simulink model "DEF_Link"  (R2018b)
settings: Solver=FixedStepDiscrete  StartTime=0.0  StopTime=10  FixedStep=0.025  RelTol=1e-3
values from neighbouring files (symbols this model uses):
  Cst_0U = uint8(0)    [DEF_ROM.m]
settings Model: Creator=CKJH7536T  LastModifiedBy=sambit.m
settings DataIOCC: LimitDataPoints=on  SaveFormat=Array  SaveOutput=off  SaveTime=off
settings OptimizationCC: DefaultParameterBehavior=Inlined  UseDivisionForNetSlopeComputation=on  UseFloatMulNetSlope=on  InlineInvariantSignals=on  EnhancedBackFolding=on  PassReuseOutputArgsAs=Individual arguments  ZeroExternalMemoryAtStartup=off  ZeroInternalMemoryAtStartup=off  NoFixptDivByZeroProtection=on  EfficientFloat2IntCast=on  OptimizeBlockOrder=speed  DifferentSizesBufferReuse=on  OptimizationCustomize=off
settings DebuggingCC: ConsistencyChecking=error  SignalInfNanChecking=error  ReadBeforeWriteMsg=EnableAllAsError  WriteAfterWriteMsg=EnableAllAsError  WriteAfterReadMsg=EnableAllAsError  AlgebraicLoopMsg=error  ArtificialAlgebraicLoopMsg=error  SaveWithDisabledLinksMsg=none  MergeDetectMultiDrivingBlocksExec=none  SignalResolutionControl=None  BlockPriorityViolationMsg=error  MinStepSizeMsg=error  TimeAdjustmentMsg=warning  SolverPrmCheckMsg=error  InheritedTsInSrcMsg=error  SingleTaskRateTransMsg=error  TasksWithSamePriorityMsg=error  SigSpecEnsureSampleTimeMsg=error  CheckMatrixSingularityMsg=error  ParameterOverflowMsg=none  ParameterPrecisionLossMsg=none  ParameterTunabilityLossMsg=error  UnderSpecifiedDataTypeMsg=warning  VectorMatrixConversionMsg=error  FcnCallInpInsideContextMsg=warning  SignalLabelMismatchMsg=warning  UnconnectedInputMsg=error  UnconnectedOutputMsg=error  UnconnectedLineMsg=error  SFcnCompatibilityMsg=error  UniqueDataStoreMsg=error  BusObjectLabelMismatch=error  RootOutportRequireBusObject=error  AssertControl=DisableAll  ModelReferenceIOMsg=error  ModelReferenceVersionMismatchMessage=error  ModelReferenceIOMismatchMessage=error  UnknownTsInhSupMsg=error  ModelReferenceDataLoggingMessage=error  StateNameClashWarn=warning  StrictBusMsg=ErrorOnBusTreatedAsVector  NonBusSignalsTreatedAsBus=error  SFInvalidInputDataAccessInChartInitDiag=error  SFTransitionOutsideNaturalParentDiag=error  SFExecutionAtInitializationDiag=none
settings HardwareCC: ProdBitPerPointer=32  ProdBitPerSizeT=32  ProdBitPerPtrDiffT=32  ProdLargestAtomicInteger=Long  ProdLargestAtomicFloat=Double  ProdWordSize=32  ProdLongLongMode=on  ProdHWDeviceType=ARM Compatible->ARM Cortex
settings ModelReferenceCC: PropagateSignalLabelsOutOfModel=off
settings SFSimCC: MATLABDynamicMemAlloc=off
settings RTWCC: SystemTargetFile=ert.tlc  GenCodeOnly=on  TemplateMakefile=ert_default_tmf  GenerateReport=on  IncludeHyperlinkInReport=on  LaunchReport=on  GenerateTraceInfo=on  GenerateTraceReport=on  GenerateTraceReportSl=on  GenerateTraceReportSf=on  GenerateTraceReportEml=on  GenerateCodeMetricsReport=on
settings CodeAppCC: ForceParamTrailComments=on  IgnoreCustomStorageClasses=off  MaxIdLength=128  OperatorAnnotations=on  SimulinkDataObjDesc=on  SFDataObjDesc=on  CustomSymbolStrGlobalVar=rt$N$M  CustomSymbolStrType=$N$M  CustomSymbolStrFcn=$N$M$F  CustomSymbolStrMacro=$N$M  InsertBlockDesc=on
settings ERTTargetCC: GenerateSampleERTMain=on  InlinedParameterPlacement=NonHierarchical  ERTCustomFileTemplate=example_file_process.tlc
settings ConfigComp: CovSaveCumulativeToWorkspaceVar=on  CovSaveSingleToWorkspaceVar=on  CovExternalEMLEnable=off

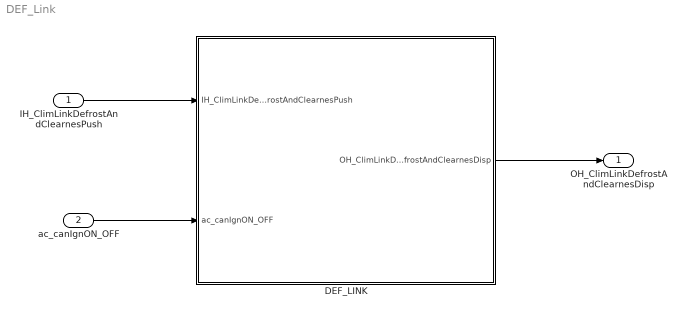
== system DEF_Link ==
  IH_ClimLinkDefrostAndClearnesPush : Inport
  ac_canIgnON_OFF : Inport  Port=2  OutDataTypeStr=boolean
  DEF_LINK : Subsystem
  OH_ClimLinkDefrostAndClearnesDisp : Outport
  wires:
  IH_ClimLinkDefrostAndClearnesPush/1 -> DEF_LINK/1(IH_ClimLinkDefrostAndClearnesPush)
  DEF_LINK/1(OH_ClimLinkDefrostAndClearnesDisp) -> OH_ClimLinkDefrostAndClearnesDisp/1
  ac_canIgnON_OFF/1 -> DEF_LINK/2(ac_canIgnON_OFF)

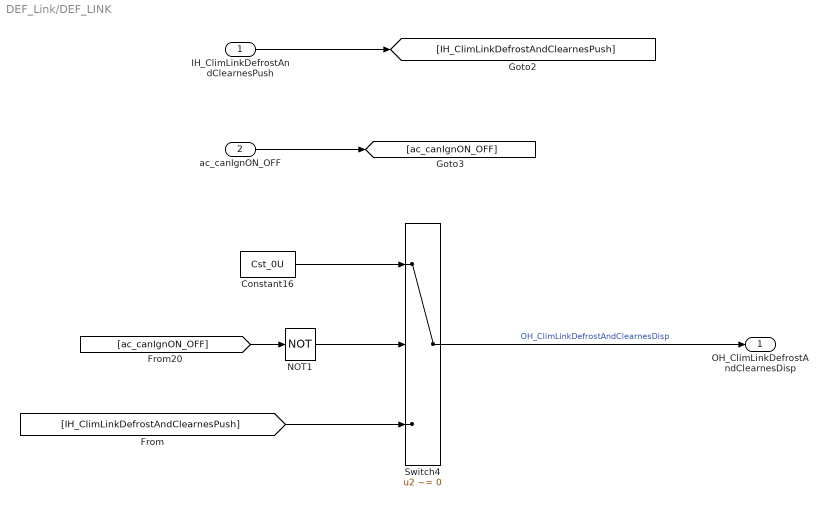
== system DEF_Link/DEF_LINK ==
  IH_ClimLinkDefrostAndClearnesPush : Inport
  ac_canIgnON_OFF : Inport  Port=2  OutDataTypeStr=boolean
  Constant16 : Constant  Value=Cst_0U
  NOT1 : Logic  Operator=NOT  AllPortsSameDT=off  OutDataTypeStr=boolean
  Switch4 : Switch  Criteria=u2 ~= 0
  OH_ClimLinkDefrostAndClearnesDisp : Outport
  wires:
  Constant16/1 -> Switch4/1
  Switch4/1 -> OH_ClimLinkDefrostAndClearnesDisp/1  "OH_ClimLinkDefrostAndClearnesDisp"
  ac_canIgnON_OFF/1 -> [ac_canIgnON_OFF]
  IH_ClimLinkDefrostAndClearnesPush/1 -> [IH_ClimLinkDefrostAndClearnesPush]
  [IH_ClimLinkDefrostAndClearnesPush] -> Switch4/3
  [ac_canIgnON_OFF] -> NOT1/1
  NOT1/1 -> Switch4/2
